simulink model "ModelLinearDig"  (R2014b)
settings: Solver=ode45  StartTime=0.0  StopTime=2  FixedStep=0.001  RelTol=1e-4
values from neighbouring files (symbols this model uses):
  H1 = Rs * (R4/R1) * 1/(R7+Rv2)    [InitModel.m]    (also in SystemModel.m = -(R4*Rs/R1) * 1/(R7+Rv2))
  R6 = 100e3    (= 100000)    [InitModel.m]    (also in SystemModel.m; SystemModel_marco.m)
  rad2rpm = 60/(2*pi)    (= 9.54929658551)    [InitModel.m]    (also in SystemModel.m)
  Vdc = 30    [InitModel.m]    (also in SystemModel.m; SystemModel_marco.m)
undefined symbols (not defined in the file or in its folder): motor
libraries: cstblocks x5
settings Model: Creator=Edoardo  LastModifiedBy=marco

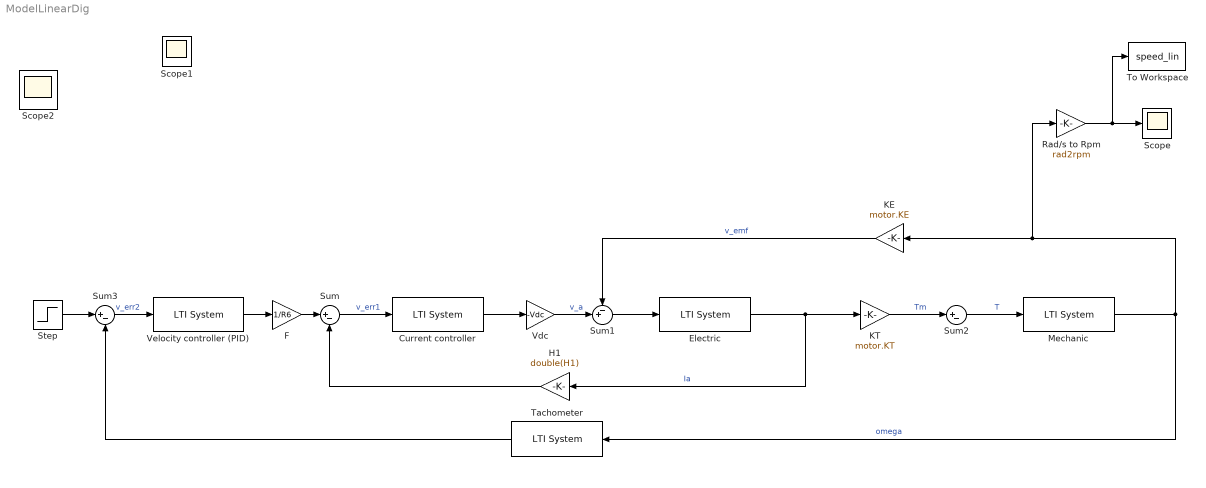
== system ModelLinearDig ==
  Current controller : cstblocks/LTI System  sys=C1_dig  IC=[]
  Electric : cstblocks/LTI System  sys=G1  IC=[]
  F : Gain  Gain=1/R6
  H1 : Gain  Gain=double(H1)
  KE : Gain  Gain=motor.KE
  KT : Gain  Gain=motor.KT
  Mechanic : cstblocks/LTI System  sys=G2  IC=[]
  Rad/s to Rpm : Gain  Gain=rad2rpm
  Scope : Scope
  Step : Step  Time=0  SampleTime=0
  Sum : Sum  Inputs=|+-
  Sum1 : Sum  Inputs=-+|
  Sum2 : Sum  Inputs=|+-
  Sum3 : Sum  Inputs=|+-
  Tachometer : cstblocks/LTI System  sys=H2  IC=[]
  To Workspace : ToWorkspace  VariableName=speed_lin  SaveFormat=Timeseries  SampleTime=-1
  Vdc : Gain  Gain=-Vdc
  Velocity controller (PID) : cstblocks/LTI System  sys=C2  IC=[]
  Scope1 : Scope
  Scope2 : Scope
      settings: SaveName=ScopeData2  MaxDataPoints=7500  Decimation=10
  wires:
  Sum1/1 -> Electric/1
  Current controller/1 -> Vdc/1
  Vdc/1 -> Sum1/2  "v_a"
  Electric/1 -> H1/1, KT/1  "Ia"
  Mechanic/1 -> KE/1, Rad/s to Rpm/1, Tachometer/1  "omega"
  KT/1 -> Sum2/1  "Tm"
  Sum2/1 -> Mechanic/1  "T"
  KE/1 -> Sum1/1  "v_emf"
  Sum/1 -> Current controller/1  "v_err1"
  H1/1 -> Sum/2
  Tachometer/1 -> Sum3/2
  Rad/s to Rpm/1 -> To Workspace/1, Scope/1
  Step/1 -> Sum3/1
  F/1 -> Sum/1
  Sum3/1 -> Velocity controller (PID)/1  "v_err2"
  Velocity controller (PID)/1 -> F/1
